simulink model "sm_tread_drive"  (R2019a)
settings: Solver=ode15s  StartTime=0.0  StopTime=50  MaxStep=0.01  RelTol=1e-4  AbsTol=1e-5  EnableMultiTasking=on
PreLoadFcn:
  | sm_tread_drive_param
StartFcn:
  | tic;
StopFcn:
  | Elapsed_Sim_Time = toc;
  | disp(['Elapsed Sim Time = ' num2str(Elapsed_Sim_Time)]);
values from neighbouring files (symbols this model uses):
  ground_sph_rad = 0.6    [sm_tread_drive_param.m]
  ground_x = 12    [sm_tread_drive_param.m]
  ground_y = 10    [sm_tread_drive_param.m]
  tread_h = tread_l/4    (= 0.7)    [sm_tread_drive_param.m]
  tread_l = 2.8    [sm_tread_drive_param.m]
  tread_rad = tread_roller_rad*1.05    (= 0.294)    [sm_tread_drive_param.m]
  tread_sep = 1.8    [sm_tread_drive_param.m]
  tread_w = 0.6    [sm_tread_drive_param.m]
undefined symbols (not defined in the file or in its folder): sigbuilder_block, X, Y, Z
libraries: sm_lib x34, Contact_Forces_Lib x14, Parts_Lib x8, fl_lib x6, nesl_utility x4
(part 2 of 2)

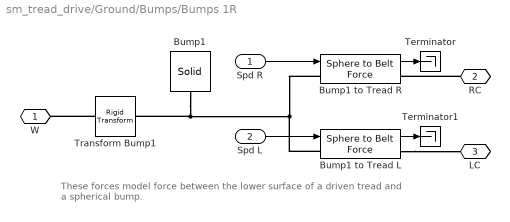
== system sm_tread_drive/Ground/Bumps/Bumps 1R ==
  note: These forces model force between the lower surface of a driven tread and a spherical bump.
  Spd R : Inport
  Spd L : Inport  Port=2
  Bump1 : sm_lib/Body Elements/Solid  InertiaType=CalculateFromGeometry  Mass=1  MassUnits=kg  CenterOfMass=[0 0 0]  CenterOfMassUnits=m  MomentsOfInertia=[1 1 1]  MomentsOfInertiaUnits=kg*m^2  ProductsOfInertia=[0 0 0]  ProductsOfInertiaUnits=kg*m^2  BasedOnType=Density  Density=1000  DensityUnits=kg/m^3  DoExposeReferenceFrame=on  SerializedFrames=<Frames/>  GraphicType=FromGeometry  MarkerShape=Sphere  MarkerSize=10  GraphicVisPropType=SimpleVisualProperties  GraphicDiffuseColor=ground_clr  GraphicSpecularColor=[0.5 0.5 0.5 1.0]  GraphicAmbientColor=[0.15 0.15 0.15 1.0]  GraphicEmissiveColor=[0.0 0.0 0.0 1.0]  GraphicShininess=75  GraphicOpacity=ground_opc  GeometryShape=Sphere  RectangleSize=[1 1]  RectangleSizeUnits=m  BrickDimensions=[1 1 1]  BrickDimensionUnits=m  CylinderRadius=1  CylinderRadiusUnits=m  CylinderLength=1  CylinderLengthUnits=m  SphereRadius=ground_sph_rad_bump  SphereRadiusUnits=m  EllipsoidRadii=[1 1 1]  EllipsoidRadiiUnits=m  ExtrusionCrossSection=[1 1; -1 1; -1 -1; 1 -1]  ExtrusionCrossSectionUnits=m  ExtrusionLength=1  ExtrusionLengthUnits=m  PolygonNumSides=3  PolygonOuterRadius=1  PolygonOuterRadiusUnits=m  ExtGeomFileType=STEP  ExtGeomFileUnits=m  RevolutionCrossSection=[1 1; 1 -1; 2 -1; 2 1]  RevolutionCrossSectionUnits=m  RevolutionExtent=Full  RevolutionAngle=180  RevolutionAngleUnits=deg
  Bump1 to Tread L : Contact_Forces_Lib/3D/Composite Forces/Sphere to Belt Force  sph_rad=ground_sph_rad_bump  belt_h=tread_rad*2  belt_w=tread_w  belt_l=tread_l  force_law_sph2bel=Linear  k_contact_sph2bel=ground_k  b_contact_sph2bel=ground_b  pen_full_damp_F_sph2bel=tread_h*1e-2  pen_exponent_sph2bel=1  friction_law_sph2bel=Stick-Slip Continuous  mu_kinetic_sph2bel=tread_muk  mu_static_sph2bel=tread_mus  v_thr_sph2bel=tread_vth  vis_on_sph2bel=off  vis_opc_en_sph2bel=0  vis_depth_sph2bel=tread_h*0.01  vis_clr=[0.9 0.2 0.2]  vis_opc=0.7
      settings: SourceProductName=Simscape Multibody Contact Forces Library
  Bump1 to Tread R : Contact_Forces_Lib/3D/Composite Forces/Sphere to Belt Force  sph_rad=ground_sph_rad_bump  belt_h=tread_rad*2  belt_w=tread_w  belt_l=tread_l  force_law_sph2bel=Linear  k_contact_sph2bel=ground_k  b_contact_sph2bel=ground_b  pen_full_damp_F_sph2bel=tread_h*1e-2  pen_exponent_sph2bel=1  friction_law_sph2bel=Stick-Slip Continuous  mu_kinetic_sph2bel=tread_muk  mu_static_sph2bel=tread_mus  v_thr_sph2bel=tread_vth  vis_on_sph2bel=off  vis_opc_en_sph2bel=0  vis_depth_sph2bel=tread_h*0.01  vis_clr=[0.9 0.2 0.2]  vis_opc=0.7
      settings: SourceProductName=Simscape Multibody Contact Forces Library
  Terminator : Terminator
  Terminator1 : Terminator
  Transform Bump1 : sm_lib/Frames and Transforms/Rigid Transform  TranslationMethod=Cartesian  TranslationStandardOffset=0  TranslationLengthUnit=m  TranslationStandardAxis=+Z  TranslationCartesianOffset=[-ground_x/2+tread_l*2 -tread_sep/2 0]  TranslationROffset=0  TranslationROffsetUnits=m  TranslationZOffset=0  TranslationZOffsetUnits=m  TranslationThetaOffset=0  TranslationThetaOffsetUnits=deg  RotationMethod=None  RotationAngleUnits=deg  RotationStandardAxis=+Z  RotationAngle=0.0  RotationArbitraryAxis=[0 0 1]  FollAlignAxisA=+X  BaseAlignAxisA=+Y  FollAlignAxisB=+Y  BaseAlignAxisB=+Z  RotationSequenceAxes=FollowerAxes  RotationSequence=XYX  RotationSequenceAngles=[0 0 0]  RotationSequenceAnglesUnits=deg  RotationMatrix=[1 0 0; 0 1 0; 0 0 1]
  W : PMIOPort  Side=Left
  RC : PMIOPort  Port=2  Side=Right
  LC : PMIOPort  Port=3  Side=Right
  wires:
  Spd R/1 -> Bump1 to Tread R/1
  Bump1 to Tread R/1 -> Terminator/1
  Spd L/1 -> Bump1 to Tread L/1
  Bump1 to Tread L/1 -> Terminator1/1
  connections:
  Bump1/RConn1 -- Bump1 to Tread L/LConn1 -- Bump1 to Tread R/LConn1 -- Transform Bump1/RConn1
  RC/RConn1 -- Bump1 to Tread R/RConn1
  Bump1 to Tread L/RConn1 -- LC/RConn1
  Transform Bump1/LConn1 -- W/RConn1

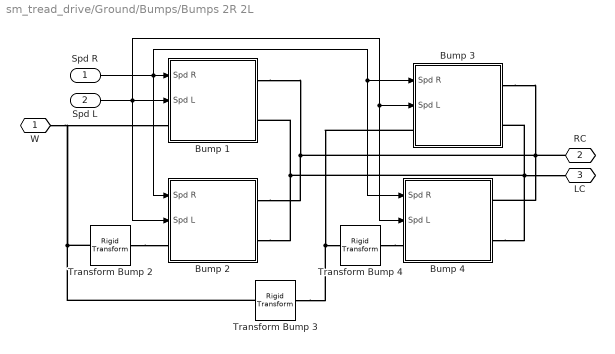
== system sm_tread_drive/Ground/Bumps/Bumps 2R 2L ==
  Spd R : Inport
  Spd L : Inport  Port=2
  Bump 1 : Subsystem
  Bump 2 : Subsystem
  Bump 3 : Subsystem
  Bump 4 : Subsystem
  Transform Bump 2 : sm_lib/Frames and Transforms/Rigid Transform  TranslationMethod=StandardAxis  TranslationStandardOffset=tread_sep  TranslationLengthUnit=m  TranslationStandardAxis=+Y  TranslationCartesianOffset=[0 0 0]  TranslationROffset=0  TranslationROffsetUnits=m  TranslationZOffset=0  TranslationZOffsetUnits=m  TranslationThetaOffset=0  TranslationThetaOffsetUnits=deg  RotationMethod=None  RotationAngleUnits=deg  RotationStandardAxis=+Z  RotationAngle=0.0  RotationArbitraryAxis=[0 0 1]  FollAlignAxisA=+X  BaseAlignAxisA=+Y  FollAlignAxisB=+Y  BaseAlignAxisB=+Z  RotationSequenceAxes=FollowerAxes  RotationSequence=XYX  RotationSequenceAngles=[0 0 0]  RotationSequenceAnglesUnits=deg  RotationMatrix=[1 0 0; 0 1 0; 0 0 1]
  Transform Bump 3 : sm_lib/Frames and Transforms/Rigid Transform  TranslationMethod=StandardAxis  TranslationStandardOffset=tread_l/3  TranslationLengthUnit=m  TranslationStandardAxis=+X  TranslationCartesianOffset=[0 0 0]  TranslationROffset=0  TranslationROffsetUnits=m  TranslationZOffset=0  TranslationZOffsetUnits=m  TranslationThetaOffset=0  TranslationThetaOffsetUnits=deg  RotationMethod=None  RotationAngleUnits=deg  RotationStandardAxis=+Z  RotationAngle=0.0  RotationArbitraryAxis=[0 0 1]  FollAlignAxisA=+X  BaseAlignAxisA=+Y  FollAlignAxisB=+Y  BaseAlignAxisB=+Z  RotationSequenceAxes=FollowerAxes  RotationSequence=XYX  RotationSequenceAngles=[0 0 0]  RotationSequenceAnglesUnits=deg  RotationMatrix=[1 0 0; 0 1 0; 0 0 1]
  Transform Bump 4 : sm_lib/Frames and Transforms/Rigid Transform  TranslationMethod=StandardAxis  TranslationStandardOffset=tread_sep  TranslationLengthUnit=m  TranslationStandardAxis=+Y  TranslationCartesianOffset=[0 0 0]  TranslationROffset=0  TranslationROffsetUnits=m  TranslationZOffset=0  TranslationZOffsetUnits=m  TranslationThetaOffset=0  TranslationThetaOffsetUnits=deg  RotationMethod=None  RotationAngleUnits=deg  RotationStandardAxis=+Z  RotationAngle=0.0  RotationArbitraryAxis=[0 0 1]  FollAlignAxisA=+X  BaseAlignAxisA=+Y  FollAlignAxisB=+Y  BaseAlignAxisB=+Z  RotationSequenceAxes=FollowerAxes  RotationSequence=XYX  RotationSequenceAngles=[0 0 0]  RotationSequenceAnglesUnits=deg  RotationMatrix=[1 0 0; 0 1 0; 0 0 1]
  W : PMIOPort  Side=Left
  RC : PMIOPort  Port=2  Side=Right
  LC : PMIOPort  Port=3  Side=Right
  wires:
  Spd L/1 -> Bump 2/2(Spd L), Bump 3/2(Spd L), Bump 4/2(Spd L), Bump 1/2(Spd L)
  Spd R/1 -> Bump 2/1(Spd R), Bump 3/1(Spd R), Bump 4/1(Spd R), Bump 1/1(Spd R)
  connections:
  Bump 3/LConn1 -- Transform Bump 3/RConn1 -- Transform Bump 4/LConn1
  Bump 3/RConn1 -- Bump 4/RConn1 -- RC/RConn1 -- Bump 2/RConn1 -- Bump 1/RConn1
  Transform Bump 2/RConn1 -- Bump 2/LConn1
  Transform Bump 3/LConn1 -- W/RConn1 -- Bump 1/LConn1 -- Transform Bump 2/LConn1
  Transform Bump 4/RConn1 -- Bump 4/LConn1
  Bump 4/RConn2 -- Bump 2/RConn2 -- Bump 1/RConn2 -- LC/RConn1 -- Bump 3/RConn2

== system sm_tread_drive/Ground/Bumps/Bumps None ==
  Spd R : Inport
  Spd L : Inport  Port=2
  Terminator1 : Terminator
  Terminator2 : Terminator
  W : PMIOPort  Side=Left
  RC : PMIOPort  Port=2  Side=Right
  LC : PMIOPort  Port=3  Side=Right
  wires:
  Spd L/1 -> Terminator1/1
  Spd R/1 -> Terminator2/1

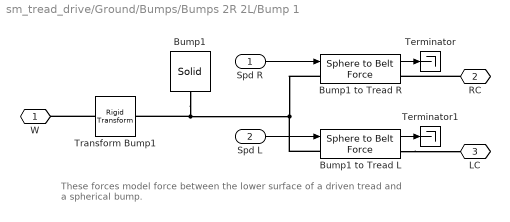
== system sm_tread_drive/Ground/Bumps/Bumps 2R 2L/Bump 1 ==
  note: These forces model force between the lower surface of a driven tread and a spherical bump.
  Spd R : Inport
  Spd L : Inport  Port=2
  Bump1 : sm_lib/Body Elements/Solid  InertiaType=CalculateFromGeometry  Mass=1  MassUnits=kg  CenterOfMass=[0 0 0]  CenterOfMassUnits=m  MomentsOfInertia=[1 1 1]  MomentsOfInertiaUnits=kg*m^2  ProductsOfInertia=[0 0 0]  ProductsOfInertiaUnits=kg*m^2  BasedOnType=Density  Density=1000  DensityUnits=kg/m^3  DoExposeReferenceFrame=on  SerializedFrames=<Frames/>  GraphicType=FromGeometry  MarkerShape=Sphere  MarkerSize=10  GraphicVisPropType=SimpleVisualProperties  GraphicDiffuseColor=ground_clr  GraphicSpecularColor=[0.5 0.5 0.5 1.0]  GraphicAmbientColor=[0.15 0.15 0.15 1.0]  GraphicEmissiveColor=[0.0 0.0 0.0 1.0]  GraphicShininess=75  GraphicOpacity=ground_opc  GeometryShape=Sphere  RectangleSize=[1 1]  RectangleSizeUnits=m  BrickDimensions=[1 1 1]  BrickDimensionUnits=m  CylinderRadius=1  CylinderRadiusUnits=m  CylinderLength=1  CylinderLengthUnits=m  SphereRadius=ground_sph_rad_bump  SphereRadiusUnits=m  EllipsoidRadii=[1 1 1]  EllipsoidRadiiUnits=m  ExtrusionCrossSection=[1 1; -1 1; -1 -1; 1 -1]  ExtrusionCrossSectionUnits=m  ExtrusionLength=1  ExtrusionLengthUnits=m  PolygonNumSides=3  PolygonOuterRadius=1  PolygonOuterRadiusUnits=m  ExtGeomFileType=STEP  ExtGeomFileUnits=m  RevolutionCrossSection=[1 1; 1 -1; 2 -1; 2 1]  RevolutionCrossSectionUnits=m  RevolutionExtent=Full  RevolutionAngle=180  RevolutionAngleUnits=deg
  Bump1 to Tread L : Contact_Forces_Lib/3D/Composite Forces/Sphere to Belt Force  sph_rad=ground_sph_rad_bump  belt_h=tread_rad*2  belt_w=tread_w  belt_l=tread_l  force_law_sph2bel=Linear  k_contact_sph2bel=ground_k  b_contact_sph2bel=ground_b  pen_full_damp_F_sph2bel=tread_h*1e-2  pen_exponent_sph2bel=1  friction_law_sph2bel=Stick-Slip Continuous  mu_kinetic_sph2bel=tread_muk  mu_static_sph2bel=tread_mus  v_thr_sph2bel=tread_vth  vis_on_sph2bel=off  vis_opc_en_sph2bel=0  vis_depth_sph2bel=tread_h*0.01  vis_clr=[0.9 0.2 0.2]  vis_opc=0.7
      settings: SourceProductName=Simscape Multibody Contact Forces Library
  Bump1 to Tread R : Contact_Forces_Lib/3D/Composite Forces/Sphere to Belt Force  sph_rad=ground_sph_rad_bump  belt_h=tread_rad*2  belt_w=tread_w  belt_l=tread_l  force_law_sph2bel=Linear  k_contact_sph2bel=ground_k  b_contact_sph2bel=ground_b  pen_full_damp_F_sph2bel=tread_h*1e-2  pen_exponent_sph2bel=1  friction_law_sph2bel=Stick-Slip Continuous  mu_kinetic_sph2bel=tread_muk  mu_static_sph2bel=tread_mus  v_thr_sph2bel=tread_vth  vis_on_sph2bel=off  vis_opc_en_sph2bel=0  vis_depth_sph2bel=tread_h*0.01  vis_clr=[0.9 0.2 0.2]  vis_opc=0.7
      settings: SourceProductName=Simscape Multibody Contact Forces Library
  Terminator : Terminator
  Terminator1 : Terminator
  Transform Bump1 : sm_lib/Frames and Transforms/Rigid Transform  TranslationMethod=Cartesian  TranslationStandardOffset=0  TranslationLengthUnit=m  TranslationStandardAxis=+Z  TranslationCartesianOffset=[-ground_x/2+tread_l*2 -tread_sep/2 0]  TranslationROffset=0  TranslationROffsetUnits=m  TranslationZOffset=0  TranslationZOffsetUnits=m  TranslationThetaOffset=0  TranslationThetaOffsetUnits=deg  RotationMethod=None  RotationAngleUnits=deg  RotationStandardAxis=+Z  RotationAngle=0.0  RotationArbitraryAxis=[0 0 1]  FollAlignAxisA=+X  BaseAlignAxisA=+Y  FollAlignAxisB=+Y  BaseAlignAxisB=+Z  RotationSequenceAxes=FollowerAxes  RotationSequence=XYX  RotationSequenceAngles=[0 0 0]  RotationSequenceAnglesUnits=deg  RotationMatrix=[1 0 0; 0 1 0; 0 0 1]
  W : PMIOPort  Side=Left
  RC : PMIOPort  Port=2  Side=Right
  LC : PMIOPort  Port=3  Side=Right
  wires:
  Spd R/1 -> Bump1 to Tread R/1
  Bump1 to Tread R/1 -> Terminator/1
  Spd L/1 -> Bump1 to Tread L/1
  Bump1 to Tread L/1 -> Terminator1/1
  connections:
  Bump1/RConn1 -- Bump1 to Tread L/LConn1 -- Bump1 to Tread R/LConn1 -- Transform Bump1/RConn1
  RC/RConn1 -- Bump1 to Tread R/RConn1
  Bump1 to Tread L/RConn1 -- LC/RConn1
  Transform Bump1/LConn1 -- W/RConn1

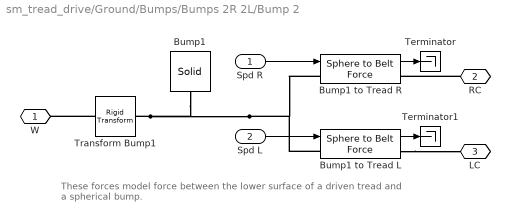
== system sm_tread_drive/Ground/Bumps/Bumps 2R 2L/Bump 2 ==
  note: These forces model force between the lower surface of a driven tread and a spherical bump.
  Spd R : Inport
  Spd L : Inport  Port=2
  Bump1 : sm_lib/Body Elements/Solid  InertiaType=CalculateFromGeometry  Mass=1  MassUnits=kg  CenterOfMass=[0 0 0]  CenterOfMassUnits=m  MomentsOfInertia=[1 1 1]  MomentsOfInertiaUnits=kg*m^2  ProductsOfInertia=[0 0 0]  ProductsOfInertiaUnits=kg*m^2  BasedOnType=Density  Density=1000  DensityUnits=kg/m^3  DoExposeReferenceFrame=on  SerializedFrames=<Frames/>  GraphicType=FromGeometry  MarkerShape=Sphere  MarkerSize=10  GraphicVisPropType=SimpleVisualProperties  GraphicDiffuseColor=ground_clr  GraphicSpecularColor=[0.5 0.5 0.5 1.0]  GraphicAmbientColor=[0.15 0.15 0.15 1.0]  GraphicEmissiveColor=[0.0 0.0 0.0 1.0]  GraphicShininess=75  GraphicOpacity=ground_opc  GeometryShape=Sphere  RectangleSize=[1 1]  RectangleSizeUnits=m  BrickDimensions=[1 1 1]  BrickDimensionUnits=m  CylinderRadius=1  CylinderRadiusUnits=m  CylinderLength=1  CylinderLengthUnits=m  SphereRadius=ground_sph_rad_bump  SphereRadiusUnits=m  EllipsoidRadii=[1 1 1]  EllipsoidRadiiUnits=m  ExtrusionCrossSection=[1 1; -1 1; -1 -1; 1 -1]  ExtrusionCrossSectionUnits=m  ExtrusionLength=1  ExtrusionLengthUnits=m  PolygonNumSides=3  PolygonOuterRadius=1  PolygonOuterRadiusUnits=m  ExtGeomFileType=STEP  ExtGeomFileUnits=m  RevolutionCrossSection=[1 1; 1 -1; 2 -1; 2 1]  RevolutionCrossSectionUnits=m  RevolutionExtent=Full  RevolutionAngle=180  RevolutionAngleUnits=deg
  Bump1 to Tread L : Contact_Forces_Lib/3D/Composite Forces/Sphere to Belt Force  sph_rad=ground_sph_rad_bump  belt_h=tread_rad*2  belt_w=tread_w  belt_l=tread_l  force_law_sph2bel=Linear  k_contact_sph2bel=ground_k  b_contact_sph2bel=ground_b  pen_full_damp_F_sph2bel=tread_h*1e-2  pen_exponent_sph2bel=1  friction_law_sph2bel=Stick-Slip Continuous  mu_kinetic_sph2bel=tread_muk  mu_static_sph2bel=tread_mus  v_thr_sph2bel=tread_vth  vis_on_sph2bel=off  vis_opc_en_sph2bel=0  vis_depth_sph2bel=tread_h*0.01  vis_clr=[0.9 0.2 0.2]  vis_opc=0.7
      settings: SourceProductName=Simscape Multibody Contact Forces Library
  Bump1 to Tread R : Contact_Forces_Lib/3D/Composite Forces/Sphere to Belt Force  sph_rad=ground_sph_rad_bump  belt_h=tread_rad*2  belt_w=tread_w  belt_l=tread_l  force_law_sph2bel=Linear  k_contact_sph2bel=ground_k  b_contact_sph2bel=ground_b  pen_full_damp_F_sph2bel=tread_h*1e-2  pen_exponent_sph2bel=1  friction_law_sph2bel=Stick-Slip Continuous  mu_kinetic_sph2bel=tread_muk  mu_static_sph2bel=tread_mus  v_thr_sph2bel=tread_vth  vis_on_sph2bel=off  vis_opc_en_sph2bel=0  vis_depth_sph2bel=tread_h*0.01  vis_clr=[0.9 0.2 0.2]  vis_opc=0.7
      settings: SourceProductName=Simscape Multibody Contact Forces Library
  Terminator : Terminator
  Terminator1 : Terminator
  Transform Bump1 : sm_lib/Frames and Transforms/Rigid Transform  TranslationMethod=Cartesian  TranslationStandardOffset=0  TranslationLengthUnit=m  TranslationStandardAxis=+Z  TranslationCartesianOffset=[-ground_x/2+tread_l*2 -tread_sep/2 0]  TranslationROffset=0  TranslationROffsetUnits=m  TranslationZOffset=0  TranslationZOffsetUnits=m  TranslationThetaOffset=0  TranslationThetaOffsetUnits=deg  RotationMethod=None  RotationAngleUnits=deg  RotationStandardAxis=+Z  RotationAngle=0.0  RotationArbitraryAxis=[0 0 1]  FollAlignAxisA=+X  BaseAlignAxisA=+Y  FollAlignAxisB=+Y  BaseAlignAxisB=+Z  RotationSequenceAxes=FollowerAxes  RotationSequence=XYX  RotationSequenceAngles=[0 0 0]  RotationSequenceAnglesUnits=deg  RotationMatrix=[1 0 0; 0 1 0; 0 0 1]
  W : PMIOPort  Side=Left
  RC : PMIOPort  Port=2  Side=Right
  LC : PMIOPort  Port=3  Side=Right
  wires:
  Bump1 to Tread L/1 -> Terminator1/1
  Spd L/1 -> Bump1 to Tread L/1
  Bump1 to Tread R/1 -> Terminator/1
  Spd R/1 -> Bump1 to Tread R/1
  connections:
  Transform Bump1/LConn1 -- W/RConn1
  Bump1 to Tread L/RConn1 -- LC/RConn1
  RC/RConn1 -- Bump1 to Tread R/RConn1
  Transform Bump1/RConn1 -- Bump1 to Tread R/LConn1 -- Bump1 to Tread L/LConn1 -- Bump1/RConn1

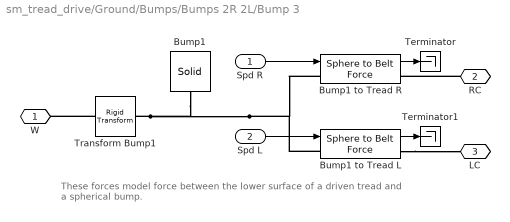
== system sm_tread_drive/Ground/Bumps/Bumps 2R 2L/Bump 3 ==
  note: These forces model force between the lower surface of a driven tread and a spherical bump.
  Spd R : Inport
  Spd L : Inport  Port=2
  Bump1 : sm_lib/Body Elements/Solid  InertiaType=CalculateFromGeometry  Mass=1  MassUnits=kg  CenterOfMass=[0 0 0]  CenterOfMassUnits=m  MomentsOfInertia=[1 1 1]  MomentsOfInertiaUnits=kg*m^2  ProductsOfInertia=[0 0 0]  ProductsOfInertiaUnits=kg*m^2  BasedOnType=Density  Density=1000  DensityUnits=kg/m^3  DoExposeReferenceFrame=on  SerializedFrames=<Frames/>  GraphicType=FromGeometry  MarkerShape=Sphere  MarkerSize=10  GraphicVisPropType=SimpleVisualProperties  GraphicDiffuseColor=ground_clr  GraphicSpecularColor=[0.5 0.5 0.5 1.0]  GraphicAmbientColor=[0.15 0.15 0.15 1.0]  GraphicEmissiveColor=[0.0 0.0 0.0 1.0]  GraphicShininess=75  GraphicOpacity=ground_opc  GeometryShape=Sphere  RectangleSize=[1 1]  RectangleSizeUnits=m  BrickDimensions=[1 1 1]  BrickDimensionUnits=m  CylinderRadius=1  CylinderRadiusUnits=m  CylinderLength=1  CylinderLengthUnits=m  SphereRadius=ground_sph_rad_bump  SphereRadiusUnits=m  EllipsoidRadii=[1 1 1]  EllipsoidRadiiUnits=m  ExtrusionCrossSection=[1 1; -1 1; -1 -1; 1 -1]  ExtrusionCrossSectionUnits=m  ExtrusionLength=1  ExtrusionLengthUnits=m  PolygonNumSides=3  PolygonOuterRadius=1  PolygonOuterRadiusUnits=m  ExtGeomFileType=STEP  ExtGeomFileUnits=m  RevolutionCrossSection=[1 1; 1 -1; 2 -1; 2 1]  RevolutionCrossSectionUnits=m  RevolutionExtent=Full  RevolutionAngle=180  RevolutionAngleUnits=deg
  Bump1 to Tread L : Contact_Forces_Lib/3D/Composite Forces/Sphere to Belt Force  sph_rad=ground_sph_rad_bump  belt_h=tread_rad*2  belt_w=tread_w  belt_l=tread_l  force_law_sph2bel=Linear  k_contact_sph2bel=ground_k  b_contact_sph2bel=ground_b  pen_full_damp_F_sph2bel=tread_h*1e-2  pen_exponent_sph2bel=1  friction_law_sph2bel=Stick-Slip Continuous  mu_kinetic_sph2bel=tread_muk  mu_static_sph2bel=tread_mus  v_thr_sph2bel=tread_vth  vis_on_sph2bel=off  vis_opc_en_sph2bel=0  vis_depth_sph2bel=tread_h*0.01  vis_clr=[0.9 0.2 0.2]  vis_opc=0.7
      settings: SourceProductName=Simscape Multibody Contact Forces Library
  Bump1 to Tread R : Contact_Forces_Lib/3D/Composite Forces/Sphere to Belt Force  sph_rad=ground_sph_rad_bump  belt_h=tread_rad*2  belt_w=tread_w  belt_l=tread_l  force_law_sph2bel=Linear  k_contact_sph2bel=ground_k  b_contact_sph2bel=ground_b  pen_full_damp_F_sph2bel=tread_h*1e-2  pen_exponent_sph2bel=1  friction_law_sph2bel=Stick-Slip Continuous  mu_kinetic_sph2bel=tread_muk  mu_static_sph2bel=tread_mus  v_thr_sph2bel=tread_vth  vis_on_sph2bel=off  vis_opc_en_sph2bel=0  vis_depth_sph2bel=tread_h*0.01  vis_clr=[0.9 0.2 0.2]  vis_opc=0.7
      settings: SourceProductName=Simscape Multibody Contact Forces Library
  Terminator : Terminator
  Terminator1 : Terminator
  Transform Bump1 : sm_lib/Frames and Transforms/Rigid Transform  TranslationMethod=Cartesian  TranslationStandardOffset=0  TranslationLengthUnit=m  TranslationStandardAxis=+Z  TranslationCartesianOffset=[-ground_x/2+tread_l*2 -tread_sep/2 0]  TranslationROffset=0  TranslationROffsetUnits=m  TranslationZOffset=0  TranslationZOffsetUnits=m  TranslationThetaOffset=0  TranslationThetaOffsetUnits=deg  RotationMethod=None  RotationAngleUnits=deg  RotationStandardAxis=+Z  RotationAngle=0.0  RotationArbitraryAxis=[0 0 1]  FollAlignAxisA=+X  BaseAlignAxisA=+Y  FollAlignAxisB=+Y  BaseAlignAxisB=+Z  RotationSequenceAxes=FollowerAxes  RotationSequence=XYX  RotationSequenceAngles=[0 0 0]  RotationSequenceAnglesUnits=deg  RotationMatrix=[1 0 0; 0 1 0; 0 0 1]
  W : PMIOPort  Side=Left
  RC : PMIOPort  Port=2  Side=Right
  LC : PMIOPort  Port=3  Side=Right
  wires:
  Bump1 to Tread L/1 -> Terminator1/1
  Spd L/1 -> Bump1 to Tread L/1
  Bump1 to Tread R/1 -> Terminator/1
  Spd R/1 -> Bump1 to Tread R/1
  connections:
  Transform Bump1/LConn1 -- W/RConn1
  Bump1 to Tread L/RConn1 -- LC/RConn1
  RC/RConn1 -- Bump1 to Tread R/RConn1
  Transform Bump1/RConn1 -- Bump1 to Tread R/LConn1 -- Bump1 to Tread L/LConn1 -- Bump1/RConn1

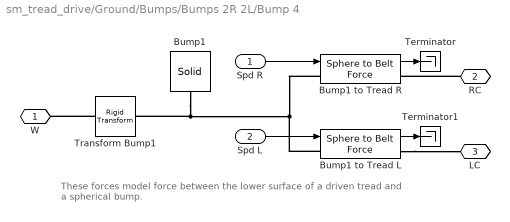
== system sm_tread_drive/Ground/Bumps/Bumps 2R 2L/Bump 4 ==
  note: These forces model force between the lower surface of a driven tread and a spherical bump.
  Spd R : Inport
  Spd L : Inport  Port=2
  Bump1 : sm_lib/Body Elements/Solid  InertiaType=CalculateFromGeometry  Mass=1  MassUnits=kg  CenterOfMass=[0 0 0]  CenterOfMassUnits=m  MomentsOfInertia=[1 1 1]  MomentsOfInertiaUnits=kg*m^2  ProductsOfInertia=[0 0 0]  ProductsOfInertiaUnits=kg*m^2  BasedOnType=Density  Density=1000  DensityUnits=kg/m^3  DoExposeReferenceFrame=on  SerializedFrames=<Frames/>  GraphicType=FromGeometry  MarkerShape=Sphere  MarkerSize=10  GraphicVisPropType=SimpleVisualProperties  GraphicDiffuseColor=ground_clr  GraphicSpecularColor=[0.5 0.5 0.5 1.0]  GraphicAmbientColor=[0.15 0.15 0.15 1.0]  GraphicEmissiveColor=[0.0 0.0 0.0 1.0]  GraphicShininess=75  GraphicOpacity=ground_opc  GeometryShape=Sphere  RectangleSize=[1 1]  RectangleSizeUnits=m  BrickDimensions=[1 1 1]  BrickDimensionUnits=m  CylinderRadius=1  CylinderRadiusUnits=m  CylinderLength=1  CylinderLengthUnits=m  SphereRadius=ground_sph_rad_bump  SphereRadiusUnits=m  EllipsoidRadii=[1 1 1]  EllipsoidRadiiUnits=m  ExtrusionCrossSection=[1 1; -1 1; -1 -1; 1 -1]  ExtrusionCrossSectionUnits=m  ExtrusionLength=1  ExtrusionLengthUnits=m  PolygonNumSides=3  PolygonOuterRadius=1  PolygonOuterRadiusUnits=m  ExtGeomFileType=STEP  ExtGeomFileUnits=m  RevolutionCrossSection=[1 1; 1 -1; 2 -1; 2 1]  RevolutionCrossSectionUnits=m  RevolutionExtent=Full  RevolutionAngle=180  RevolutionAngleUnits=deg
  Bump1 to Tread L : Contact_Forces_Lib/3D/Composite Forces/Sphere to Belt Force  sph_rad=ground_sph_rad_bump  belt_h=tread_rad*2  belt_w=tread_w  belt_l=tread_l  force_law_sph2bel=Linear  k_contact_sph2bel=ground_k  b_contact_sph2bel=ground_b  pen_full_damp_F_sph2bel=tread_h*1e-2  pen_exponent_sph2bel=1  friction_law_sph2bel=Stick-Slip Continuous  mu_kinetic_sph2bel=tread_muk  mu_static_sph2bel=tread_mus  v_thr_sph2bel=tread_vth  vis_on_sph2bel=off  vis_opc_en_sph2bel=0  vis_depth_sph2bel=tread_h*0.01  vis_clr=[0.9 0.2 0.2]  vis_opc=0.7
      settings: SourceProductName=Simscape Multibody Contact Forces Library
  Bump1 to Tread R : Contact_Forces_Lib/3D/Composite Forces/Sphere to Belt Force  sph_rad=ground_sph_rad_bump  belt_h=tread_rad*2  belt_w=tread_w  belt_l=tread_l  force_law_sph2bel=Linear  k_contact_sph2bel=ground_k  b_contact_sph2bel=ground_b  pen_full_damp_F_sph2bel=tread_h*1e-2  pen_exponent_sph2bel=1  friction_law_sph2bel=Stick-Slip Continuous  mu_kinetic_sph2bel=tread_muk  mu_static_sph2bel=tread_mus  v_thr_sph2bel=tread_vth  vis_on_sph2bel=off  vis_opc_en_sph2bel=0  vis_depth_sph2bel=tread_h*0.01  vis_clr=[0.9 0.2 0.2]  vis_opc=0.7
      settings: SourceProductName=Simscape Multibody Contact Forces Library
  Terminator : Terminator
  Terminator1 : Terminator
  Transform Bump1 : sm_lib/Frames and Transforms/Rigid Transform  TranslationMethod=Cartesian  TranslationStandardOffset=0  TranslationLengthUnit=m  TranslationStandardAxis=+Z  TranslationCartesianOffset=[-ground_x/2+tread_l*2 -tread_sep/2 0]  TranslationROffset=0  TranslationROffsetUnits=m  TranslationZOffset=0  TranslationZOffsetUnits=m  TranslationThetaOffset=0  TranslationThetaOffsetUnits=deg  RotationMethod=None  RotationAngleUnits=deg  RotationStandardAxis=+Z  RotationAngle=0.0  RotationArbitraryAxis=[0 0 1]  FollAlignAxisA=+X  BaseAlignAxisA=+Y  FollAlignAxisB=+Y  BaseAlignAxisB=+Z  RotationSequenceAxes=FollowerAxes  RotationSequence=XYX  RotationSequenceAngles=[0 0 0]  RotationSequenceAnglesUnits=deg  RotationMatrix=[1 0 0; 0 1 0; 0 0 1]
  W : PMIOPort  Side=Left
  RC : PMIOPort  Port=2  Side=Right
  LC : PMIOPort  Port=3  Side=Right
  wires:
  Spd R/1 -> Bump1 to Tread R/1
  Bump1 to Tread R/1 -> Terminator/1
  Spd L/1 -> Bump1 to Tread L/1
  Bump1 to Tread L/1 -> Terminator1/1
  connections:
  Bump1/RConn1 -- Bump1 to Tread L/LConn1 -- Bump1 to Tread R/LConn1 -- Transform Bump1/RConn1
  RC/RConn1 -- Bump1 to Tread R/RConn1
  Bump1 to Tread L/RConn1 -- LC/RConn1
  Transform Bump1/LConn1 -- W/RConn1
